simulink library "TYPEB_MASTER"  (Simulink 8.6)
settings: Solver=ode45  StartTime=0.0  StopTime=10.0  RelTol=1e-3
libraries: cdsEpicsOut x19, STATE_BIO_MASTER x17, cdsEpicsBinIn x15, cdsBit2Word x12, GAS_MASTER x12, cdsWord2Bit x5, cdsEpicsStringIn x4, cdsDacKill x4, ISC_common x4, IP_MASTER x4, cdsFilt x4, cdsEpicsMomentary x4
(part 2 of 3)

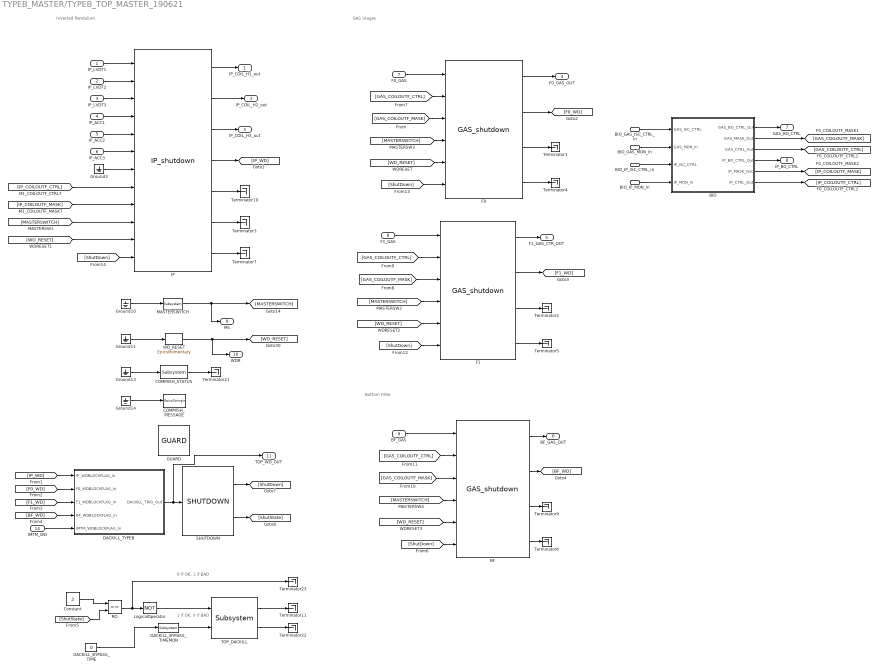
== system TYPEB_MASTER/TYPEB_TOP_MASTER_190621 ==
  note: Inverted Pendulum
  note: GAS Stages
  note: Bottom Filter
  note: 0 if OK, 1 if BAD
  note: 1 if OK, 0 if BAD
  IP_LVDT1 : Inport
  IP_LVDT2 : Inport  Port=2
  IP_LVDT3 : Inport  Port=3
  IP_ACC1 : Inport  Port=4
  IP_ACC2 : Inport  Port=5
  IP_ACC3 : Inport  Port=6
  F0_GAS : Inport  Port=7
  F1_GAS : Inport  Port=8
  BF_GAS : Inport  Port=9
  BIO_GAS_ISC_CTRL_In : Inport  Port=10
  BIO_GAS_MON_In : Inport  Port=11
  BIO_IP_ISC_CTRL_In : Inport  Port=12
  BIO_IP_MON_In : Inport  Port=13
  IMTM_WD : Inport  Port=14
  BF : GAS_MASTER/GAS_shutdown
  BIO : Subsystem
  COMMISH_MESSAGE : cdsEpicsStringIn/EpicsStringIn  Tag=cdsEpicsStringIn  Description=cdsEpicsStringIn
      settings: AttributesFormatString=%<Tag>
  COMMISH_STATUS : cdsEpicsBinIn/Subsystem  Tag=cdsEpicsBinIn  Description=|
      | Purpose:                                                                            
      | Create an EPICS binary (0 or 1) input channel to the FE realtime controls.          
      |                                                                                     
      | Operation:                                                                          
      | Outputs value from an EPICS ai record. Value is binary input (bi Epics record type).
      |                                                                                     
      | Usage:                                                                              
      | Name the part with the desired EPICS channel name.
      settings: AttributesFormatString=%<Tag>
  Constant : Constant  Value=2
  DACKILL_BYPASS_TIME : Constant  Value=0
  DACKILL_BYPASS_TIMEMON : cdsEpicsOut/Subsystem  Tag=cdsEpicsOutput  Description=|
      | Purpose:                                          
      | Output a FE signal to an EPICS channel.           
      |                                                   
      | Operation:                                        
      | Takes input value and passes it to EPICS record.  
      |                                                   
      | Usage:                                            
      | Name the part with the desired EPICS rrecord name.
      settings: AttributesFormatString=%<Tag>
  DACKILL_TYPEB : Subsystem
  F0 : GAS_MASTER/GAS_shutdown
  F1 : GAS_MASTER/GAS_shutdown
  GUARD : ISC_common/GUARD
  Ground{3,10..11,13..14} (5 alike) : Ground
  IP : IP_MASTER/IP_shutdown
  LogicalOperator : Logic  Operator=NOT  AllPortsSameDT=off  OutDataTypeStr=boolean
  MASTERSWITCH : cdsEpicsBinIn/Subsystem  Tag=cdsEpicsBinIn  Description=|
      | Purpose:                                                                            
      | Create an EPICS binary (0 or 1) input channel to the FE realtime controls.          
      |                                                                                     
      | Operation:                                                                          
      | Outputs value from an EPICS ai record. Value is binary input (bi Epics record type).
      |                                                                                     
      | Usage:                                                                              
      | Name the part with the desired EPICS channel name.
      settings: AttributesFormatString=%<Tag>
  RO : RelationalOperator  Operator===  OutDataTypeStr=boolean
  SHUTDOWN : SHUTDOWN/SHUTDOWN
  TOP_DACKILL : cdsDacKill/Subsystem  Description=cdsDacKill
      settings: AttributesFormatString=%<Description>
  Terminator{1..7,9..11,21..23} (13 alike) : Terminator
  WD_RESET : cdsEpicsMomentary/EpicsMomentary  Tag=cdsEpicsMomentary
      settings: AttributesFormatString=%<Tag>
  IP_COIL_H1_out : Outport
  IP_COIL_H2_out : Outport  Port=2
  IP_COIL_H3_out : Outport  Port=3
  F0_GAS_OUT : Outport  Port=4
  F1_GAS_CTR_OUT : Outport  Port=5
  BF_GAS_OUT : Outport  Port=6
  GAS_BO_CTRL : Outport  Port=7
  IP_BO_CTRL : Outport  Port=8
  MS : Outport  Port=9
  WDR : Outport  Port=10
  TOP_WD_OUT : Outport  Port=11
  wires:
  F1_GAS/1 -> F1/1
  [GAS_COILOUTF_MASK] -> F0/3
  [GAS_COILOUTF_CTRL] -> F0/2
  [GAS_COILOUTF_CTRL] -> BF/2
  [MASTERSWITCH] -> F0/4
  [GAS_COILOUTF_MASK] -> BF/3
  [IP_COILOUTF_CTRL] -> IP/8
  BIO/6(IP_CTRL_Out) -> [IP_COILOUTF_CTRL]
  [MASTERSWITCH] -> BF/4
  BF/1 -> BF_GAS_OUT/1
  IP_LVDT1/1 -> IP/1
  F1/1 -> F1_GAS_CTR_OUT/1
  BIO/3(GAS_CTRL_Out) -> [GAS_COILOUTF_CTRL]
  BIO/5(IP_MASK_Out) -> [IP_COILOUTF_MASK]
  F1/3 -> Terminator2/1
  LogicalOperator/1 -> TOP_DACKILL/1
  [WD_RESET] -> F1/5
  IP_LVDT2/1 -> IP/2
  [MASTERSWITCH] -> IP/10
  Ground3/1 -> IP/7
  F0/3 -> Terminator1/1
  IP/3 -> IP_COIL_H3_out/1
  BF_GAS/1 -> BF/1
  F1/2 -> [F1_WD]
  F0_GAS/1 -> F0/1
  [MASTERSWITCH] -> F1/4
  IP_LVDT3/1 -> IP/3
  IP/4 -> [IP_WD]
  [F1_WD] -> DACKILL_TYPEB/3(F1_WDBLOCKFLAG_In)
  F0/1 -> F0_GAS_OUT/1
  Ground11/1 -> WD_RESET/1
  [BF_WD] -> DACKILL_TYPEB/4(BF_WDBLOCKFLAG_In)
  IP/2 -> IP_COIL_H2_out/1
  IP/1 -> IP_COIL_H1_out/1
  Ground10/1 -> MASTERSWITCH/1
  DACKILL_BYPASS_TIME/1 -> DACKILL_BYPASS_TIMEMON/1
  F0/2 -> [F0_WD]
  IP_ACC1/1 -> IP/4
  [WD_RESET] -> BF/5
  TOP_DACKILL/1 -> Terminator11/1
  IMTM_WD/1 -> DACKILL_TYPEB/5(IMTM_WDBLOCKFLAG_In)
  [F0_WD] -> DACKILL_TYPEB/2(F0_WDBLOCKFLAG_In)
  [GAS_COILOUTF_CTRL] -> F1/2
  IP_ACC3/1 -> IP/6
  BF/2 -> [BF_WD]
  Ground14/1 -> COMMISH_MESSAGE/1
  IP/5 -> Terminator10/1
  BF/3 -> Terminator9/1
  DACKILL_BYPASS_TIMEMON/1 -> TOP_DACKILL/2
  [WD_RESET] -> IP/11
  IP_ACC2/1 -> IP/5
  [IP_WD] -> DACKILL_TYPEB/1(IP_WDBLOCKFLAG_In)
  COMMISH_STATUS/1 -> Terminator21/1
  Ground13/1 -> COMMISH_STATUS/1
  TOP_DACKILL/2 -> Terminator22/1
  BIO/4(IP_BO_CTRL_Out) -> IP_BO_CTRL/1
  BIO/1(GAS_BO_CTRL_Out) -> GAS_BO_CTRL/1
  BIO_IP_MON_In/1 -> BIO/4(IP_MON_In)
  BIO/2(GAS_MASK_Out) -> [GAS_COILOUTF_MASK]
  BIO_GAS_MON_In/1 -> BIO/2(GAS_MON_In)
  BIO_IP_ISC_CTRL_In/1 -> BIO/3(IP_ISC_CTRL)
  BIO_GAS_ISC_CTRL_In/1 -> BIO/1(GAS_ISC_CTRL)
  [IP_COILOUTF_MASK] -> IP/9
  [GAS_COILOUTF_MASK] -> F1/3
  [WD_RESET] -> F0/5
  MASTERSWITCH/1 -> MS/1, [MASTERSWITCH]
  WD_RESET/1 -> WDR/1, [WD_RESET]
  IP/6 -> Terminator3/1
  F0/4 -> Terminator4/1
  F1/4 -> Terminator5/1
  BF/4 -> Terminator6/1
  IP/7 -> Terminator7/1
  DACKILL_TYPEB/1(DACKILL_TRIG_Out) -> TOP_WD_OUT/1, SHUTDOWN/1
  SHUTDOWN/1 -> [ShutDown]
  SHUTDOWN/2 -> [ShutState]
  Constant/1 -> RO/1
  [ShutState] -> RO/2
  RO/1 -> Terminator23/1, LogicalOperator/1
  [ShutDown] -> BF/6
  [ShutDown] -> F1/6
  [ShutDown] -> F0/6
  [ShutDown] -> IP/12

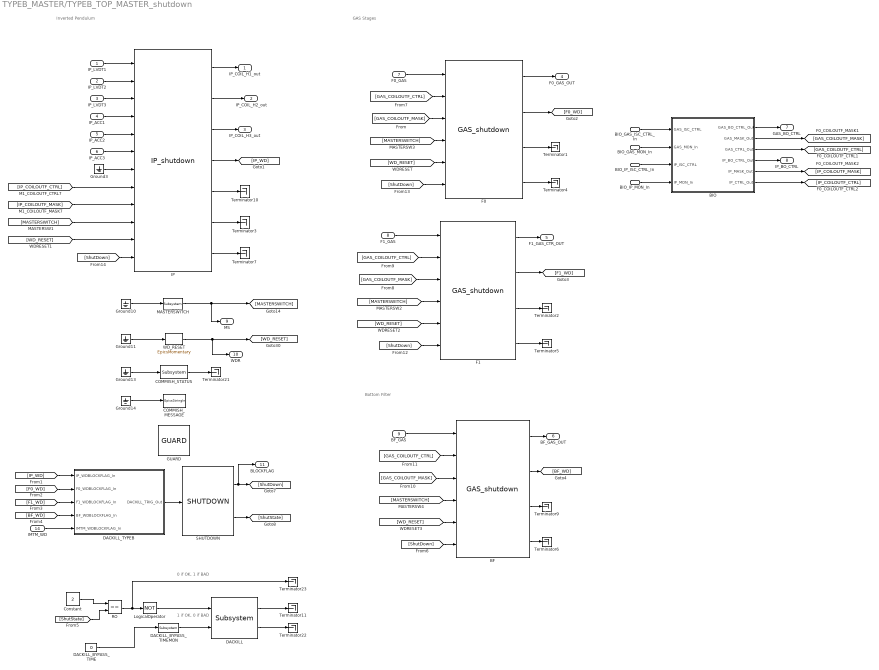
== system TYPEB_MASTER/TYPEB_TOP_MASTER_shutdown ==
  note: Inverted Pendulum
  note: GAS Stages
  note: Bottom Filter
  note: 0 if OK, 1 if BAD
  note: 1 if OK, 0 if BAD
  IP_LVDT1 : Inport
  IP_LVDT2 : Inport  Port=2
  IP_LVDT3 : Inport  Port=3
  IP_ACC1 : Inport  Port=4
  IP_ACC2 : Inport  Port=5
  IP_ACC3 : Inport  Port=6
  F0_GAS : Inport  Port=7
  F1_GAS : Inport  Port=8
  BF_GAS : Inport  Port=9
  BIO_GAS_ISC_CTRL_In : Inport  Port=10
  BIO_GAS_MON_In : Inport  Port=11
  BIO_IP_ISC_CTRL_In : Inport  Port=12
  BIO_IP_MON_In : Inport  Port=13
  IMTM_WD : Inport  Port=14
  BF : GAS_MASTER/GAS_shutdown
  BIO : Subsystem
  COMMISH_MESSAGE : cdsEpicsStringIn/EpicsStringIn  Tag=cdsEpicsStringIn  Description=cdsEpicsStringIn
      settings: AttributesFormatString=%<Tag>
  COMMISH_STATUS : cdsEpicsBinIn/Subsystem  Tag=cdsEpicsBinIn  Description=|
      | Purpose:                                                                            
      | Create an EPICS binary (0 or 1) input channel to the FE realtime controls.          
      |                                                                                     
      | Operation:                                                                          
      | Outputs value from an EPICS ai record. Value is binary input (bi Epics record type).
      |                                                                                     
      | Usage:                                                                              
      | Name the part with the desired EPICS channel name.
      settings: AttributesFormatString=%<Tag>
  Constant : Constant  Value=2
  DACKILL : cdsDacKill/Subsystem  Description=cdsDacKill
      settings: AttributesFormatString=%<Description>
  DACKILL_BYPASS_TIME : Constant  Value=0
  DACKILL_BYPASS_TIMEMON : cdsEpicsOut/Subsystem  Tag=cdsEpicsOutput  Description=|
      | Purpose:                                          
      | Output a FE signal to an EPICS channel.           
      |                                                   
      | Operation:                                        
      | Takes input value and passes it to EPICS record.  
      |                                                   
      | Usage:                                            
      | Name the part with the desired EPICS rrecord name.
      settings: AttributesFormatString=%<Tag>
  DACKILL_TYPEB : Subsystem
  F0 : GAS_MASTER/GAS_shutdown
  F1 : GAS_MASTER/GAS_shutdown
  GUARD : ISC_common/GUARD
  Ground{3,10..11,13..14} (5 alike) : Ground
  IP : IP_MASTER/IP_shutdown
  LogicalOperator : Logic  Operator=NOT  AllPortsSameDT=off  OutDataTypeStr=boolean
  MASTERSWITCH : cdsEpicsBinIn/Subsystem  Tag=cdsEpicsBinIn  Description=|
      | Purpose:                                                                            
      | Create an EPICS binary (0 or 1) input channel to the FE realtime controls.          
      |                                                                                     
      | Operation:                                                                          
      | Outputs value from an EPICS ai record. Value is binary input (bi Epics record type).
      |                                                                                     
      | Usage:                                                                              
      | Name the part with the desired EPICS channel name.
      settings: AttributesFormatString=%<Tag>
  RO : RelationalOperator  Operator===  OutDataTypeStr=boolean
  SHUTDOWN : SHUTDOWN/SHUTDOWN
  Terminator{1..7,9..11,21..23} (13 alike) : Terminator
  WD_RESET : cdsEpicsMomentary/EpicsMomentary  Tag=cdsEpicsMomentary
      settings: AttributesFormatString=%<Tag>
  IP_COIL_H1_out : Outport
  IP_COIL_H2_out : Outport  Port=2
  IP_COIL_H3_out : Outport  Port=3
  F0_GAS_OUT : Outport  Port=4
  F1_GAS_CTR_OUT : Outport  Port=5
  BF_GAS_OUT : Outport  Port=6
  GAS_BO_CTRL : Outport  Port=7
  IP_BO_CTRL : Outport  Port=8
  MS : Outport  Port=9
  WDR : Outport  Port=10
  BLOCKFLAG : Outport  Port=11
  wires:
  F1_GAS/1 -> F1/1
  [GAS_COILOUTF_MASK] -> F0/3
  [GAS_COILOUTF_CTRL] -> F0/2
  [GAS_COILOUTF_CTRL] -> BF/2
  [MASTERSWITCH] -> F0/4
  [GAS_COILOUTF_MASK] -> BF/3
  [IP_COILOUTF_CTRL] -> IP/8
  BIO/6(IP_CTRL_Out) -> [IP_COILOUTF_CTRL]
  [MASTERSWITCH] -> BF/4
  BF/1 -> BF_GAS_OUT/1
  IP_LVDT1/1 -> IP/1
  F1/1 -> F1_GAS_CTR_OUT/1
  BIO/3(GAS_CTRL_Out) -> [GAS_COILOUTF_CTRL]
  BIO/5(IP_MASK_Out) -> [IP_COILOUTF_MASK]
  F1/3 -> Terminator2/1
  LogicalOperator/1 -> DACKILL/1
  [WD_RESET] -> F1/5
  IP_LVDT2/1 -> IP/2
  [MASTERSWITCH] -> IP/10
  Ground3/1 -> IP/7
  F0/3 -> Terminator1/1
  IP/3 -> IP_COIL_H3_out/1
  BF_GAS/1 -> BF/1
  F1/2 -> [F1_WD]
  F0_GAS/1 -> F0/1
  [MASTERSWITCH] -> F1/4
  IP_LVDT3/1 -> IP/3
  IP/4 -> [IP_WD]
  [F1_WD] -> DACKILL_TYPEB/3(F1_WDBLOCKFLAG_In)
  F0/1 -> F0_GAS_OUT/1
  Ground11/1 -> WD_RESET/1
  [BF_WD] -> DACKILL_TYPEB/4(BF_WDBLOCKFLAG_In)
  IP/2 -> IP_COIL_H2_out/1
  IP/1 -> IP_COIL_H1_out/1
  Ground10/1 -> MASTERSWITCH/1
  DACKILL_BYPASS_TIME/1 -> DACKILL_BYPASS_TIMEMON/1
  F0/2 -> [F0_WD]
  IP_ACC1/1 -> IP/4
  [WD_RESET] -> BF/5
  DACKILL/1 -> Terminator11/1
  IMTM_WD/1 -> DACKILL_TYPEB/5(IMTM_WDBLOCKFLAG_In)
  [F0_WD] -> DACKILL_TYPEB/2(F0_WDBLOCKFLAG_In)
  [GAS_COILOUTF_CTRL] -> F1/2
  IP_ACC3/1 -> IP/6
  BF/2 -> [BF_WD]
  Ground14/1 -> COMMISH_MESSAGE/1
  IP/5 -> Terminator10/1
  BF/3 -> Terminator9/1
  DACKILL_BYPASS_TIMEMON/1 -> DACKILL/2
  [WD_RESET] -> IP/11
  IP_ACC2/1 -> IP/5
  [IP_WD] -> DACKILL_TYPEB/1(IP_WDBLOCKFLAG_In)
  COMMISH_STATUS/1 -> Terminator21/1
  Ground13/1 -> COMMISH_STATUS/1
  DACKILL/2 -> Terminator22/1
  BIO/4(IP_BO_CTRL_Out) -> IP_BO_CTRL/1
  BIO/1(GAS_BO_CTRL_Out) -> GAS_BO_CTRL/1
  BIO_IP_MON_In/1 -> BIO/4(IP_MON_In)
  BIO/2(GAS_MASK_Out) -> [GAS_COILOUTF_MASK]
  BIO_GAS_MON_In/1 -> BIO/2(GAS_MON_In)
  BIO_IP_ISC_CTRL_In/1 -> BIO/3(IP_ISC_CTRL)
  BIO_GAS_ISC_CTRL_In/1 -> BIO/1(GAS_ISC_CTRL)
  [IP_COILOUTF_MASK] -> IP/9
  [GAS_COILOUTF_MASK] -> F1/3
  [WD_RESET] -> F0/5
  MASTERSWITCH/1 -> MS/1, [MASTERSWITCH]
  WD_RESET/1 -> WDR/1, [WD_RESET]
  IP/6 -> Terminator3/1
  F0/4 -> Terminator4/1
  F1/4 -> Terminator5/1
  BF/4 -> Terminator6/1
  IP/7 -> Terminator7/1
  DACKILL_TYPEB/1(DACKILL_TRIG_Out) -> SHUTDOWN/1
  SHUTDOWN/1 -> BLOCKFLAG/1, [ShutDown]
  SHUTDOWN/2 -> [ShutState]
  Constant/1 -> RO/1
  [ShutState] -> RO/2
  RO/1 -> Terminator23/1, LogicalOperator/1
  [ShutDown] -> BF/6
  [ShutDown] -> F1/6
  [ShutDown] -> F0/6
  [ShutDown] -> IP/12

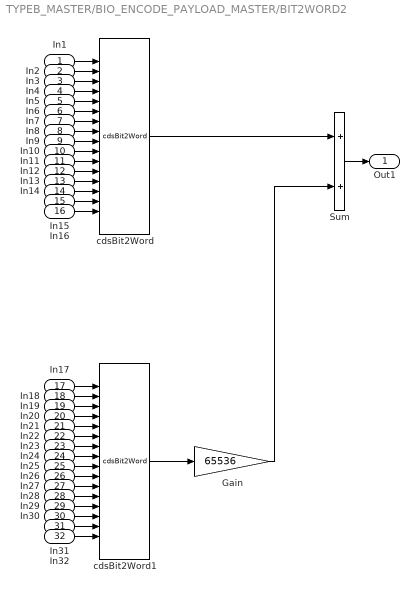
== system TYPEB_MASTER/BIO_ENCODE_PAYLOAD_MASTER/BIT2WORD2 ==
  In1 : Inport
  In2 : Inport  Port=2
  In3 : Inport  Port=3
  In4 : Inport  Port=4
  In5 : Inport  Port=5
  In6 : Inport  Port=6
  In7 : Inport  Port=7
  In8 : Inport  Port=8
  In9 : Inport  Port=9
  In10 : Inport  Port=10
  In11 : Inport  Port=11
  In12 : Inport  Port=12
  In13 : Inport  Port=13
  In14 : Inport  Port=14
  In15 : Inport  Port=15
  In16 : Inport  Port=16
  In17 : Inport  Port=17
  In18 : Inport  Port=18
  In19 : Inport  Port=19
  In20 : Inport  Port=20
  In21 : Inport  Port=21
  In22 : Inport  Port=22
  In23 : Inport  Port=23
  In24 : Inport  Port=24
  In25 : Inport  Port=25
  In26 : Inport  Port=26
  In27 : Inport  Port=27
  In28 : Inport  Port=28
  In29 : Inport  Port=29
  In30 : Inport  Port=30
  In31 : Inport  Port=31
  In32 : Inport  Port=32
  Gain : Gain  Gain=65536
  Sum : Sum
  cdsBit2Word : cdsBit2Word/cdsBit2Word  Tag=cdsBit2Word  Description=Forms single 16 bit integer from 16 0/1 inputs.
      settings: AttributesFormatString=%<Tag>
  cdsBit2Word1 : cdsBit2Word/cdsBit2Word  Tag=cdsBit2Word  Description=Forms single 16 bit integer from 16 0/1 inputs.
      settings: AttributesFormatString=%<Tag>
  Out1 : Outport
  wires:
  Gain/1 -> Sum/2
  cdsBit2Word1/1 -> Gain/1
  cdsBit2Word/1 -> Sum/1
  In1/1 -> cdsBit2Word/1
  In2/1 -> cdsBit2Word/2
  In3/1 -> cdsBit2Word/3
  In4/1 -> cdsBit2Word/4
  In5/1 -> cdsBit2Word/5
  In6/1 -> cdsBit2Word/6
  In7/1 -> cdsBit2Word/7
  In8/1 -> cdsBit2Word/8
  In9/1 -> cdsBit2Word/9
  In10/1 -> cdsBit2Word/10
  Sum/1 -> Out1/1
  In11/1 -> cdsBit2Word/11
  In12/1 -> cdsBit2Word/12
  In13/1 -> cdsBit2Word/13
  In14/1 -> cdsBit2Word/14
  In15/1 -> cdsBit2Word/15
  In16/1 -> cdsBit2Word/16
  In17/1 -> cdsBit2Word1/1
  In18/1 -> cdsBit2Word1/2
  In19/1 -> cdsBit2Word1/3
  In20/1 -> cdsBit2Word1/4
  In21/1 -> cdsBit2Word1/5
  In22/1 -> cdsBit2Word1/6
  In23/1 -> cdsBit2Word1/7
  In24/1 -> cdsBit2Word1/8
  In25/1 -> cdsBit2Word1/9
  In26/1 -> cdsBit2Word1/10
  In27/1 -> cdsBit2Word1/11
  In28/1 -> cdsBit2Word1/12
  In29/1 -> cdsBit2Word1/13
  In30/1 -> cdsBit2Word1/14
  In31/1 -> cdsBit2Word1/15
  In32/1 -> cdsBit2Word1/16

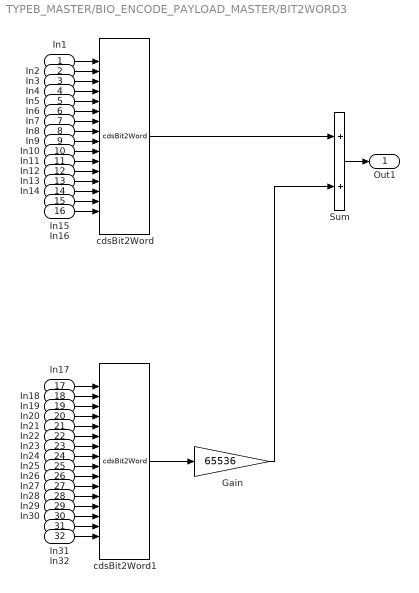
== system TYPEB_MASTER/BIO_ENCODE_PAYLOAD_MASTER/BIT2WORD3 ==
  In1 : Inport
  In2 : Inport  Port=2
  In3 : Inport  Port=3
  In4 : Inport  Port=4
  In5 : Inport  Port=5
  In6 : Inport  Port=6
  In7 : Inport  Port=7
  In8 : Inport  Port=8
  In9 : Inport  Port=9
  In10 : Inport  Port=10
  In11 : Inport  Port=11
  In12 : Inport  Port=12
  In13 : Inport  Port=13
  In14 : Inport  Port=14
  In15 : Inport  Port=15
  In16 : Inport  Port=16
  In17 : Inport  Port=17
  In18 : Inport  Port=18
  In19 : Inport  Port=19
  In20 : Inport  Port=20
  In21 : Inport  Port=21
  In22 : Inport  Port=22
  In23 : Inport  Port=23
  In24 : Inport  Port=24
  In25 : Inport  Port=25
  In26 : Inport  Port=26
  In27 : Inport  Port=27
  In28 : Inport  Port=28
  In29 : Inport  Port=29
  In30 : Inport  Port=30
  In31 : Inport  Port=31
  In32 : Inport  Port=32
  Gain : Gain  Gain=65536
  Sum : Sum
  cdsBit2Word : cdsBit2Word/cdsBit2Word  Tag=cdsBit2Word  Description=Forms single 16 bit integer from 16 0/1 inputs.
      settings: AttributesFormatString=%<Tag>
  cdsBit2Word1 : cdsBit2Word/cdsBit2Word  Tag=cdsBit2Word  Description=Forms single 16 bit integer from 16 0/1 inputs.
      settings: AttributesFormatString=%<Tag>
  Out1 : Outport
  wires:
  Gain/1 -> Sum/2
  cdsBit2Word1/1 -> Gain/1
  cdsBit2Word/1 -> Sum/1
  In1/1 -> cdsBit2Word/1
  In2/1 -> cdsBit2Word/2
  In3/1 -> cdsBit2Word/3
  In4/1 -> cdsBit2Word/4
  In5/1 -> cdsBit2Word/5
  In6/1 -> cdsBit2Word/6
  In7/1 -> cdsBit2Word/7
  In8/1 -> cdsBit2Word/8
  In9/1 -> cdsBit2Word/9
  In10/1 -> cdsBit2Word/10
  Sum/1 -> Out1/1
  In11/1 -> cdsBit2Word/11
  In12/1 -> cdsBit2Word/12
  In13/1 -> cdsBit2Word/13
  In14/1 -> cdsBit2Word/14
  In15/1 -> cdsBit2Word/15
  In16/1 -> cdsBit2Word/16
  In17/1 -> cdsBit2Word1/1
  In18/1 -> cdsBit2Word1/2
  In19/1 -> cdsBit2Word1/3
  In20/1 -> cdsBit2Word1/4
  In21/1 -> cdsBit2Word1/5
  In22/1 -> cdsBit2Word1/6
  In23/1 -> cdsBit2Word1/7
  In24/1 -> cdsBit2Word1/8
  In25/1 -> cdsBit2Word1/9
  In26/1 -> cdsBit2Word1/10
  In27/1 -> cdsBit2Word1/11
  In28/1 -> cdsBit2Word1/12
  In29/1 -> cdsBit2Word1/13
  In30/1 -> cdsBit2Word1/14
  In31/1 -> cdsBit2Word1/15
  In32/1 -> cdsBit2Word1/16

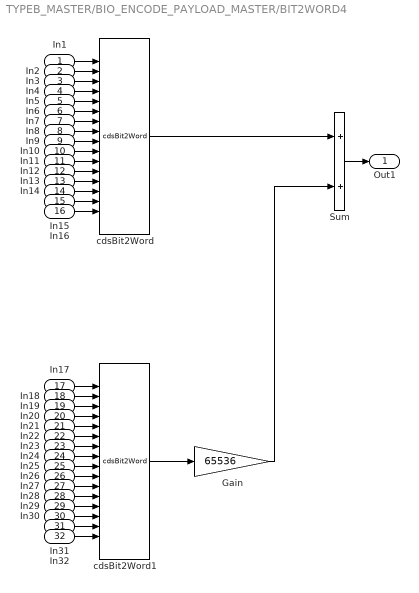
== system TYPEB_MASTER/BIO_ENCODE_PAYLOAD_MASTER/BIT2WORD4 ==
  In1 : Inport
  In2 : Inport  Port=2
  In3 : Inport  Port=3
  In4 : Inport  Port=4
  In5 : Inport  Port=5
  In6 : Inport  Port=6
  In7 : Inport  Port=7
  In8 : Inport  Port=8
  In9 : Inport  Port=9
  In10 : Inport  Port=10
  In11 : Inport  Port=11
  In12 : Inport  Port=12
  In13 : Inport  Port=13
  In14 : Inport  Port=14
  In15 : Inport  Port=15
  In16 : Inport  Port=16
  In17 : Inport  Port=17
  In18 : Inport  Port=18
  In19 : Inport  Port=19
  In20 : Inport  Port=20
  In21 : Inport  Port=21
  In22 : Inport  Port=22
  In23 : Inport  Port=23
  In24 : Inport  Port=24
  In25 : Inport  Port=25
  In26 : Inport  Port=26
  In27 : Inport  Port=27
  In28 : Inport  Port=28
  In29 : Inport  Port=29
  In30 : Inport  Port=30
  In31 : Inport  Port=31
  In32 : Inport  Port=32
  Gain : Gain  Gain=65536
  Sum : Sum
  cdsBit2Word : cdsBit2Word/cdsBit2Word  Tag=cdsBit2Word  Description=Forms single 16 bit integer from 16 0/1 inputs.
      settings: AttributesFormatString=%<Tag>
  cdsBit2Word1 : cdsBit2Word/cdsBit2Word  Tag=cdsBit2Word  Description=Forms single 16 bit integer from 16 0/1 inputs.
      settings: AttributesFormatString=%<Tag>
  Out1 : Outport
  wires:
  Gain/1 -> Sum/2
  cdsBit2Word1/1 -> Gain/1
  cdsBit2Word/1 -> Sum/1
  In1/1 -> cdsBit2Word/1
  In2/1 -> cdsBit2Word/2
  In3/1 -> cdsBit2Word/3
  In4/1 -> cdsBit2Word/4
  In5/1 -> cdsBit2Word/5
  In6/1 -> cdsBit2Word/6
  In7/1 -> cdsBit2Word/7
  In8/1 -> cdsBit2Word/8
  In9/1 -> cdsBit2Word/9
  In10/1 -> cdsBit2Word/10
  Sum/1 -> Out1/1
  In11/1 -> cdsBit2Word/11
  In12/1 -> cdsBit2Word/12
  In13/1 -> cdsBit2Word/13
  In14/1 -> cdsBit2Word/14
  In15/1 -> cdsBit2Word/15
  In16/1 -> cdsBit2Word/16
  In17/1 -> cdsBit2Word1/1
  In18/1 -> cdsBit2Word1/2
  In19/1 -> cdsBit2Word1/3
  In20/1 -> cdsBit2Word1/4
  In21/1 -> cdsBit2Word1/5
  In22/1 -> cdsBit2Word1/6
  In23/1 -> cdsBit2Word1/7
  In24/1 -> cdsBit2Word1/8
  In25/1 -> cdsBit2Word1/9
  In26/1 -> cdsBit2Word1/10
  In27/1 -> cdsBit2Word1/11
  In28/1 -> cdsBit2Word1/12
  In29/1 -> cdsBit2Word1/13
  In30/1 -> cdsBit2Word1/14
  In31/1 -> cdsBit2Word1/15
  In32/1 -> cdsBit2Word1/16

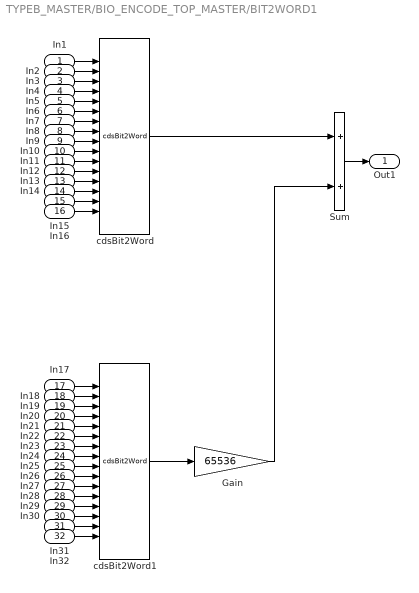
== system TYPEB_MASTER/BIO_ENCODE_TOP_MASTER/BIT2WORD1 ==
  In1 : Inport
  In2 : Inport  Port=2
  In3 : Inport  Port=3
  In4 : Inport  Port=4
  In5 : Inport  Port=5
  In6 : Inport  Port=6
  In7 : Inport  Port=7
  In8 : Inport  Port=8
  In9 : Inport  Port=9
  In10 : Inport  Port=10
  In11 : Inport  Port=11
  In12 : Inport  Port=12
  In13 : Inport  Port=13
  In14 : Inport  Port=14
  In15 : Inport  Port=15
  In16 : Inport  Port=16
  In17 : Inport  Port=17
  In18 : Inport  Port=18
  In19 : Inport  Port=19
  In20 : Inport  Port=20
  In21 : Inport  Port=21
  In22 : Inport  Port=22
  In23 : Inport  Port=23
  In24 : Inport  Port=24
  In25 : Inport  Port=25
  In26 : Inport  Port=26
  In27 : Inport  Port=27
  In28 : Inport  Port=28
  In29 : Inport  Port=29
  In30 : Inport  Port=30
  In31 : Inport  Port=31
  In32 : Inport  Port=32
  Gain : Gain  Gain=65536
  Sum : Sum
  cdsBit2Word : cdsBit2Word/cdsBit2Word  Tag=cdsBit2Word  Description=Forms single 16 bit integer from 16 0/1 inputs.
      settings: AttributesFormatString=%<Tag>
  cdsBit2Word1 : cdsBit2Word/cdsBit2Word  Tag=cdsBit2Word  Description=Forms single 16 bit integer from 16 0/1 inputs.
      settings: AttributesFormatString=%<Tag>
  Out1 : Outport
  wires:
  Gain/1 -> Sum/2
  cdsBit2Word1/1 -> Gain/1
  cdsBit2Word/1 -> Sum/1
  In1/1 -> cdsBit2Word/1
  In2/1 -> cdsBit2Word/2
  In3/1 -> cdsBit2Word/3
  In4/1 -> cdsBit2Word/4
  In5/1 -> cdsBit2Word/5
  In6/1 -> cdsBit2Word/6
  In7/1 -> cdsBit2Word/7
  In8/1 -> cdsBit2Word/8
  In9/1 -> cdsBit2Word/9
  In10/1 -> cdsBit2Word/10
  Sum/1 -> Out1/1
  In11/1 -> cdsBit2Word/11
  In12/1 -> cdsBit2Word/12
  In13/1 -> cdsBit2Word/13
  In14/1 -> cdsBit2Word/14
  In15/1 -> cdsBit2Word/15
  In16/1 -> cdsBit2Word/16
  In17/1 -> cdsBit2Word1/1
  In18/1 -> cdsBit2Word1/2
  In19/1 -> cdsBit2Word1/3
  In20/1 -> cdsBit2Word1/4
  In21/1 -> cdsBit2Word1/5
  In22/1 -> cdsBit2Word1/6
  In23/1 -> cdsBit2Word1/7
  In24/1 -> cdsBit2Word1/8
  In25/1 -> cdsBit2Word1/9
  In26/1 -> cdsBit2Word1/10
  In27/1 -> cdsBit2Word1/11
  In28/1 -> cdsBit2Word1/12
  In29/1 -> cdsBit2Word1/13
  In30/1 -> cdsBit2Word1/14
  In31/1 -> cdsBit2Word1/15
  In32/1 -> cdsBit2Word1/16

== system TYPEB_MASTER/BIO_ENCODE_TOP_MASTER/BIT2WORD2 ==
  In1 : Inport
  In2 : Inport  Port=2
  In3 : Inport  Port=3
  In4 : Inport  Port=4
  In5 : Inport  Port=5
  In6 : Inport  Port=6
  In7 : Inport  Port=7
  In8 : Inport  Port=8
  In9 : Inport  Port=9
  In10 : Inport  Port=10
  In11 : Inport  Port=11
  In12 : Inport  Port=12
  In13 : Inport  Port=13
  In14 : Inport  Port=14
  In15 : Inport  Port=15
  In16 : Inport  Port=16
  In17 : Inport  Port=17
  In18 : Inport  Port=18
  In19 : Inport  Port=19
  In20 : Inport  Port=20
  In21 : Inport  Port=21
  In22 : Inport  Port=22
  In23 : Inport  Port=23
  In24 : Inport  Port=24
  In25 : Inport  Port=25
  In26 : Inport  Port=26
  In27 : Inport  Port=27
  In28 : Inport  Port=28
  In29 : Inport  Port=29
  In30 : Inport  Port=30
  In31 : Inport  Port=31
  In32 : Inport  Port=32
  Gain : Gain  Gain=65536
  Sum : Sum
  cdsBit2Word : cdsBit2Word/cdsBit2Word  Tag=cdsBit2Word  Description=Forms single 16 bit integer from 16 0/1 inputs.
      settings: AttributesFormatString=%<Tag>
  cdsBit2Word1 : cdsBit2Word/cdsBit2Word  Tag=cdsBit2Word  Description=Forms single 16 bit integer from 16 0/1 inputs.
      settings: AttributesFormatString=%<Tag>
  Out1 : Outport
  wires:
  Gain/1 -> Sum/2
  cdsBit2Word1/1 -> Gain/1
  cdsBit2Word/1 -> Sum/1
  In1/1 -> cdsBit2Word/1
  In2/1 -> cdsBit2Word/2
  In3/1 -> cdsBit2Word/3
  In4/1 -> cdsBit2Word/4
  In5/1 -> cdsBit2Word/5
  In6/1 -> cdsBit2Word/6
  In7/1 -> cdsBit2Word/7
  In8/1 -> cdsBit2Word/8
  In9/1 -> cdsBit2Word/9
  In10/1 -> cdsBit2Word/10
  Sum/1 -> Out1/1
  In11/1 -> cdsBit2Word/11
  In12/1 -> cdsBit2Word/12
  In13/1 -> cdsBit2Word/13
  In14/1 -> cdsBit2Word/14
  In15/1 -> cdsBit2Word/15
  In16/1 -> cdsBit2Word/16
  In17/1 -> cdsBit2Word1/1
  In18/1 -> cdsBit2Word1/2
  In19/1 -> cdsBit2Word1/3
  In20/1 -> cdsBit2Word1/4
  In21/1 -> cdsBit2Word1/5
  In22/1 -> cdsBit2Word1/6
  In23/1 -> cdsBit2Word1/7
  In24/1 -> cdsBit2Word1/8
  In25/1 -> cdsBit2Word1/9
  In26/1 -> cdsBit2Word1/10
  In27/1 -> cdsBit2Word1/11
  In28/1 -> cdsBit2Word1/12
  In29/1 -> cdsBit2Word1/13
  In30/1 -> cdsBit2Word1/14
  In31/1 -> cdsBit2Word1/15
  In32/1 -> cdsBit2Word1/16

== system TYPEB_MASTER/BIO_ENCODE_TOP_MASTER/BIT2WORD5 ==
  In1 : Inport
  In2 : Inport  Port=2
  In3 : Inport  Port=3
  In4 : Inport  Port=4
  In5 : Inport  Port=5
  In6 : Inport  Port=6
  In7 : Inport  Port=7
  In8 : Inport  Port=8
  In9 : Inport  Port=9
  In10 : Inport  Port=10
  In11 : Inport  Port=11
  In12 : Inport  Port=12
  In13 : Inport  Port=13
  In14 : Inport  Port=14
  In15 : Inport  Port=15
  In16 : Inport  Port=16
  In17 : Inport  Port=17
  In18 : Inport  Port=18
  In19 : Inport  Port=19
  In20 : Inport  Port=20
  In21 : Inport  Port=21
  In22 : Inport  Port=22
  In23 : Inport  Port=23
  In24 : Inport  Port=24
  In25 : Inport  Port=25
  In26 : Inport  Port=26
  In27 : Inport  Port=27
  In28 : Inport  Port=28
  In29 : Inport  Port=29
  In30 : Inport  Port=30
  In31 : Inport  Port=31
  In32 : Inport  Port=32
  Gain : Gain  Gain=65536
  Sum : Sum
  cdsBit2Word : cdsBit2Word/cdsBit2Word  Tag=cdsBit2Word  Description=Forms single 16 bit integer from 16 0/1 inputs.
      settings: AttributesFormatString=%<Tag>
  cdsBit2Word1 : cdsBit2Word/cdsBit2Word  Tag=cdsBit2Word  Description=Forms single 16 bit integer from 16 0/1 inputs.
      settings: AttributesFormatString=%<Tag>
  Out1 : Outport
  wires:
  Gain/1 -> Sum/2
  cdsBit2Word1/1 -> Gain/1
  cdsBit2Word/1 -> Sum/1
  In1/1 -> cdsBit2Word/1
  In2/1 -> cdsBit2Word/2
  In3/1 -> cdsBit2Word/3
  In4/1 -> cdsBit2Word/4
  In5/1 -> cdsBit2Word/5
  In6/1 -> cdsBit2Word/6
  In7/1 -> cdsBit2Word/7
  In8/1 -> cdsBit2Word/8
  In9/1 -> cdsBit2Word/9
  In10/1 -> cdsBit2Word/10
  Sum/1 -> Out1/1
  In11/1 -> cdsBit2Word/11
  In12/1 -> cdsBit2Word/12
  In13/1 -> cdsBit2Word/13
  In14/1 -> cdsBit2Word/14
  In15/1 -> cdsBit2Word/15
  In16/1 -> cdsBit2Word/16
  In17/1 -> cdsBit2Word1/1
  In18/1 -> cdsBit2Word1/2
  In19/1 -> cdsBit2Word1/3
  In20/1 -> cdsBit2Word1/4
  In21/1 -> cdsBit2Word1/5
  In22/1 -> cdsBit2Word1/6
  In23/1 -> cdsBit2Word1/7
  In24/1 -> cdsBit2Word1/8
  In25/1 -> cdsBit2Word1/9
  In26/1 -> cdsBit2Word1/10
  In27/1 -> cdsBit2Word1/11
  In28/1 -> cdsBit2Word1/12
  In29/1 -> cdsBit2Word1/13
  In30/1 -> cdsBit2Word1/14
  In31/1 -> cdsBit2Word1/15
  In32/1 -> cdsBit2Word1/16

== system TYPEB_MASTER/TYPEB_MASTER/BIO ==
  note: 12 Bit Word
  note: 12 Bit Word
  note: 12 Bit Word
  note: 12 Bit Word
  TM_ISC_CTRL : Inport
  TM_MON_In : Inport  Port=2
  IM1_CTRL : Inport  Port=3
  IM1_MON_In : Inport  Port=4
  IM2_ISC_CTRL : Inport  Port=5
  IM2_MON_In : Inport  Port=6
  GAS_ISC_CTRL : Inport  Port=7
  GAS_MON_In : Inport  Port=8
  IP_ISC_CTRL : Inport  Port=9
  IP_MON_In : Inport  Port=10
  GAS : STATE_BIO_MASTER/UIM_BIO_MASTER
  IM1 : STATE_BIO_MASTER/UIM_BIO_MASTER
  IM2 : STATE_BIO_MASTER/UIM_BIO_MASTER
  IP : STATE_BIO_MASTER/TACQ_BIO_MASTER
  TM : STATE_BIO_MASTER/UIM_BIO_MASTER
  TM_BO_CTRL_Out : Outport
  TM_MASK_Out : Outport  Port=2
  TM_CTRL_Out : Outport  Port=3
  IM1_BO_CTRL_Out : Outport  Port=4
  IM1_MASK_Out : Outport  Port=5
  IM1_CTRL_Out : Outport  Port=6
  IM2_BO_CTRL_Out : Outport  Port=7
  IM2_MASK_Out : Outport  Port=8
  IM2_CTRL_Out : Outport  Port=9
  GAS_BO_CTRL_Out : Outport  Port=10
  GAS_MASK_Out : Outport  Port=11
  GAS_CTRL_Out : Outport  Port=12
  IP_BO_CTRL_Out : Outport  Port=13
  IP_MASK_Out : Outport  Port=14
  IP_CTRL_Out : Outport  Port=15
  wires:
  TM_MON_In/1 -> TM/2
  TM_ISC_CTRL/1 -> TM/1
  IM1_CTRL/1 -> IM1/1
  IM1_MON_In/1 -> IM1/2
  IM2_MON_In/1 -> IM2/2
  IM2_ISC_CTRL/1 -> IM2/1
  GAS_MON_In/1 -> GAS/2
  GAS_ISC_CTRL/1 -> GAS/1
  IP_MON_In/1 -> IP/2
  IP_ISC_CTRL/1 -> IP/1
  TM/1 -> TM_MASK_Out/1
  TM/2 -> TM_CTRL_Out/1
  TM/3 -> TM_BO_CTRL_Out/1
  IM1/1 -> IM1_MASK_Out/1
  IM1/2 -> IM1_CTRL_Out/1
  IM1/3 -> IM1_BO_CTRL_Out/1
  IM2/1 -> IM2_MASK_Out/1
  IM2/2 -> IM2_CTRL_Out/1
  IM2/3 -> IM2_BO_CTRL_Out/1
  GAS/1 -> GAS_MASK_Out/1
  GAS/2 -> GAS_CTRL_Out/1
  GAS/3 -> GAS_BO_CTRL_Out/1
  IP/1 -> IP_MASK_Out/1
  IP/2 -> IP_CTRL_Out/1
  IP/3 -> IP_BO_CTRL_Out/1

== system TYPEB_MASTER/TYPEB_MASTER/TM_OSEM ==
  OSEM_H1_In : Inport
  OSEM_H2_In : Inport  Port=2
  OSEM_H3_In : Inport  Port=3
  OSEM_H4_In : Inport  Port=4
  2EUL : cdsMuxMatrix/Subsystem  Tag=cdsMuxMatrix  Description=Any size matrix. Inputs and outputs must be connected using Mux and Demux parts.
      settings: AttributesFormatString=%<Tag>
  DAMP : Subsystem  AncestorBlock=SIXOSEM_F_STAGE_MASTER/SIXOSEM_F_STAGE_MASTER/DAMP
  Demux1 : Demux  Outputs=3
  Demux2 : Demux  Outputs=3
  INF : Subsystem  AncestorBlock=SIXOSEM_F_STAGE_MASTER/SIXOSEM_F_STAGE_MASTER/OSEMINF
  Mux1 : Mux  Inputs=3
  Mux2 : Mux
  SENSALIGN : cdsMuxMatrix/Subsystem  Tag=cdsMuxMatrix  Description=Any size matrix. Inputs and outputs must be connected using Mux and Demux parts.
      settings: AttributesFormatString=%<Tag>
  wires:
  Mux1/1 -> SENSALIGN/1
  SENSALIGN/1 -> Demux2/1
  Demux1/3 -> Mux1/3
  Mux2/1 -> 2EUL/1
  2EUL/1 -> Demux1/1
  Demux1/1 -> Mux1/1
  Demux1/2 -> Mux1/2
  OSEM_H1_In/1 -> INF/1(H1_In)
  OSEM_H4_In/1 -> INF/4(H4_In)
  OSEM_H3_In/1 -> INF/3(H3_In)
  OSEM_H2_In/1 -> INF/2(H2_In)
  Demux2/1 -> DAMP/1(LONG_In)
  Demux2/2 -> DAMP/2(PITCH_In)
  Demux2/3 -> DAMP/3(YAW_In)
  INF/1(H4_Out) -> Mux2/1
  INF/2(H1_Out) -> Mux2/2
  INF/3(H2_Out) -> Mux2/3
  INF/4(H3_Out) -> Mux2/4

== system TYPEB_MASTER/TYPEB_PAYLOAD_MASTER/BIO ==
  note: 12 Bit Word
  note: 12 Bit Word
  TM_ISC_CTRL : Inport
  TM_MON_In : Inport  Port=2
  IMV_CTRL : Inport  Port=3
  IMV_MON_In : Inport  Port=4
  IMH_ISC_CTRL : Inport  Port=5
  IMH_MON_In : Inport  Port=6
  IMH : STATE_BIO_MASTER/UIM_BIO_MASTER
  IMV : STATE_BIO_MASTER/UIM_BIO_MASTER
  TM : STATE_BIO_MASTER/UIM_BIO_MASTER
  TM_BO_CTRL_Out : Outport
  TM_MASK_Out : Outport  Port=2
  TM_CTRL_Out : Outport  Port=3
  IMV_BO_CTRL_Out : Outport  Port=4
  IMV_MASK_Out : Outport  Port=5
  IMV_CTRL_Out : Outport  Port=6
  IMH_BO_CTRL_Out : Outport  Port=7
  IMH_MASK_Out : Outport  Port=8
  IMH_CTRL_Out : Outport  Port=9
  wires:
  IMH/3 -> IMH_BO_CTRL_Out/1
  IMH/2 -> IMH_CTRL_Out/1
  IMH/1 -> IMH_MASK_Out/1
  IMV/3 -> IMV_BO_CTRL_Out/1
  IMV/1 -> IMV_MASK_Out/1
  IMV/2 -> IMV_CTRL_Out/1
  TM/2 -> TM_CTRL_Out/1
  TM/3 -> TM_BO_CTRL_Out/1
  TM/1 -> TM_MASK_Out/1
  IMH_ISC_CTRL/1 -> IMH/1
  IMV_MON_In/1 -> IMV/2
  IMH_MON_In/1 -> IMH/2
  TM_ISC_CTRL/1 -> TM/1
  IMV_CTRL/1 -> IMV/1
  TM_MON_In/1 -> TM/2

== system TYPEB_MASTER/TYPEB_PAYLOAD_shutdown/BIO ==
  note: 12 Bit Word
  note: 12 Bit Word
  TM_ISC_CTRL : Inport
  TM_MON_In : Inport  Port=2
  IMV_CTRL : Inport  Port=3
  IMV_MON_In : Inport  Port=4
  IMH_ISC_CTRL : Inport  Port=5
  IMH_MON_In : Inport  Port=6
  IMH : STATE_BIO_MASTER/UIM_BIO_MASTER
  IMV : STATE_BIO_MASTER/UIM_BIO_MASTER
  TM : STATE_BIO_MASTER/UIM_BIO_MASTER
  TM_BO_CTRL_Out : Outport
  TM_MASK_Out : Outport  Port=2
  TM_CTRL_Out : Outport  Port=3
  IMV_BO_CTRL_Out : Outport  Port=4
  IMV_MASK_Out : Outport  Port=5
  IMV_CTRL_Out : Outport  Port=6
  IMH_BO_CTRL_Out : Outport  Port=7
  IMH_MASK_Out : Outport  Port=8
  IMH_CTRL_Out : Outport  Port=9
  wires:
  TM_MON_In/1 -> TM/2
  IMV_CTRL/1 -> IMV/1
  TM_ISC_CTRL/1 -> TM/1
  IMH_MON_In/1 -> IMH/2
  IMV_MON_In/1 -> IMV/2
  IMH_ISC_CTRL/1 -> IMH/1
  TM/1 -> TM_MASK_Out/1
  TM/3 -> TM_BO_CTRL_Out/1
  TM/2 -> TM_CTRL_Out/1
  IMV/2 -> IMV_CTRL_Out/1
  IMV/1 -> IMV_MASK_Out/1
  IMV/3 -> IMV_BO_CTRL_Out/1
  IMH/1 -> IMH_MASK_Out/1
  IMH/2 -> IMH_CTRL_Out/1
  IMH/3 -> IMH_BO_CTRL_Out/1

== system TYPEB_MASTER/TYPEB_TOP_MASTER/BIO ==
  note: 12 Bit Word
  note: 12 Bit Word
  GAS_ISC_CTRL : Inport
  GAS_MON_In : Inport  Port=2
  IP_ISC_CTRL : Inport  Port=3
  IP_MON_In : Inport  Port=4
  GAS : STATE_BIO_MASTER/UIM_BIO_MASTER
  IP : STATE_BIO_MASTER/TACQ_BIO_MASTER
  GAS_BO_CTRL_Out : Outport
  GAS_MASK_Out : Outport  Port=2
  GAS_CTRL_Out : Outport  Port=3
  IP_BO_CTRL_Out : Outport  Port=4
  IP_MASK_Out : Outport  Port=5
  IP_CTRL_Out : Outport  Port=6
  wires:
  IP/2 -> IP_CTRL_Out/1
  GAS/1 -> GAS_MASK_Out/1
  IP_MON_In/1 -> IP/2
  IP/3 -> IP_BO_CTRL_Out/1
  GAS/2 -> GAS_CTRL_Out/1
  GAS/3 -> GAS_BO_CTRL_Out/1
  GAS_MON_In/1 -> GAS/2
  GAS_ISC_CTRL/1 -> GAS/1
  IP/1 -> IP_MASK_Out/1
  IP_ISC_CTRL/1 -> IP/1

== system TYPEB_MASTER/TYPEB_TOP_MASTER/DACKILL_TYPEB ==
  note: AND is zero  (0) if all stages are OK
      | non-zero if BAD
  note: WDBLOCKFLAG is zero (0) if OK,
      | non-zero if BAD
  IP_WDBLOCKFLAG_In : Inport
  F0_WDBLOCKFLAG_In : Inport  Port=2
  F1_WDBLOCKFLAG_In : Inport  Port=3
  BF_WDBLOCKFLAG_In : Inport  Port=4
  IMTM_WDBLOCKFLAG_In : Inport  Port=5
  LogicalOperator1 : Logic  Operator=OR  Inputs=5  AllPortsSameDT=off  OutDataTypeStr=boolean
  STATE : cdsEpicsOut/Subsystem  Tag=cdsEpicsOutput  Description=|
      | Purpose:                                          
      | Output a FE signal to an EPICS channel.           
      |                                                   
      | Operation:                                        
      | Takes input value and passes it to EPICS record.  
      |                                                   
      | Usage:                                            
      | Name the part with the desired EPICS rrecord name.
      settings: AttributesFormatString=%<Tag>
  DACKILL_TRIG_Out : Outport
  wires:
  BF_WDBLOCKFLAG_In/1 -> LogicalOperator1/4
  IMTM_WDBLOCKFLAG_In/1 -> LogicalOperator1/5
  LogicalOperator1/1 -> STATE/1
  F1_WDBLOCKFLAG_In/1 -> LogicalOperator1/3
  F0_WDBLOCKFLAG_In/1 -> LogicalOperator1/2
  IP_WDBLOCKFLAG_In/1 -> LogicalOperator1/1
  STATE/1 -> DACKILL_TRIG_Out/1

== system TYPEB_MASTER/TYPEB_TOP_MASTER_190621/BIO ==
  note: 12 Bit Word
  note: 12 Bit Word
  GAS_ISC_CTRL : Inport
  GAS_MON_In : Inport  Port=2
  IP_ISC_CTRL : Inport  Port=3
  IP_MON_In : Inport  Port=4
  GAS : STATE_BIO_MASTER/UIM_BIO_MASTER
  IP : STATE_BIO_MASTER/TACQ_BIO_MASTER
  GAS_BO_CTRL_Out : Outport
  GAS_MASK_Out : Outport  Port=2
  GAS_CTRL_Out : Outport  Port=3
  IP_BO_CTRL_Out : Outport  Port=4
  IP_MASK_Out : Outport  Port=5
  IP_CTRL_Out : Outport  Port=6
  wires:
  IP/2 -> IP_CTRL_Out/1
  GAS/1 -> GAS_MASK_Out/1
  IP_MON_In/1 -> IP/2
  IP/3 -> IP_BO_CTRL_Out/1
  GAS/2 -> GAS_CTRL_Out/1
  GAS/3 -> GAS_BO_CTRL_Out/1
  GAS_MON_In/1 -> GAS/2
  GAS_ISC_CTRL/1 -> GAS/1
  IP/1 -> IP_MASK_Out/1
  IP_ISC_CTRL/1 -> IP/1

== system TYPEB_MASTER/TYPEB_TOP_MASTER_190621/DACKILL_TYPEB ==
  note: AND is zero  (0) if all stages are OK
      | non-zero if BAD
  note: WDBLOCKFLAG is zero (0) if OK,
      | non-zero if BAD
  IP_WDBLOCKFLAG_In : Inport
  F0_WDBLOCKFLAG_In : Inport  Port=2
  F1_WDBLOCKFLAG_In : Inport  Port=3
  BF_WDBLOCKFLAG_In : Inport  Port=4
  IMTM_WDBLOCKFLAG_In : Inport  Port=5
  LogicalOperator1 : Logic  Operator=OR  Inputs=5  AllPortsSameDT=off  OutDataTypeStr=boolean
  STATE : cdsEpicsOut/Subsystem  Tag=cdsEpicsOutput  Description=|
      | Purpose:                                          
      | Output a FE signal to an EPICS channel.           
      |                                                   
      | Operation:                                        
      | Takes input value and passes it to EPICS record.  
      |                                                   
      | Usage:                                            
      | Name the part with the desired EPICS rrecord name.
      settings: AttributesFormatString=%<Tag>
  DACKILL_TRIG_Out : Outport
  wires:
  BF_WDBLOCKFLAG_In/1 -> LogicalOperator1/4
  IMTM_WDBLOCKFLAG_In/1 -> LogicalOperator1/5
  LogicalOperator1/1 -> STATE/1
  F1_WDBLOCKFLAG_In/1 -> LogicalOperator1/3
  F0_WDBLOCKFLAG_In/1 -> LogicalOperator1/2
  IP_WDBLOCKFLAG_In/1 -> LogicalOperator1/1
  STATE/1 -> DACKILL_TRIG_Out/1

== system TYPEB_MASTER/TYPEB_TOP_MASTER_shutdown/BIO ==
  note: 12 Bit Word
  note: 12 Bit Word
  GAS_ISC_CTRL : Inport
  GAS_MON_In : Inport  Port=2
  IP_ISC_CTRL : Inport  Port=3
  IP_MON_In : Inport  Port=4
  GAS : STATE_BIO_MASTER/UIM_BIO_MASTER
  IP : STATE_BIO_MASTER/TACQ_BIO_MASTER
  GAS_BO_CTRL_Out : Outport
  GAS_MASK_Out : Outport  Port=2
  GAS_CTRL_Out : Outport  Port=3
  IP_BO_CTRL_Out : Outport  Port=4
  IP_MASK_Out : Outport  Port=5
  IP_CTRL_Out : Outport  Port=6
  wires:
  IP/2 -> IP_CTRL_Out/1
  GAS/1 -> GAS_MASK_Out/1
  IP_MON_In/1 -> IP/2
  IP/3 -> IP_BO_CTRL_Out/1
  GAS/2 -> GAS_CTRL_Out/1
  GAS/3 -> GAS_BO_CTRL_Out/1
  GAS_MON_In/1 -> GAS/2
  GAS_ISC_CTRL/1 -> GAS/1
  IP/1 -> IP_MASK_Out/1
  IP_ISC_CTRL/1 -> IP/1

== system TYPEB_MASTER/TYPEB_TOP_MASTER_shutdown/DACKILL_TYPEB ==
  note: AND is zero  (0) if all stages are OK
      | non-zero if BAD
  note: WDBLOCKFLAG is zero (0) if OK,
      | non-zero if BAD
  IP_WDBLOCKFLAG_In : Inport
  F0_WDBLOCKFLAG_In : Inport  Port=2
  F1_WDBLOCKFLAG_In : Inport  Port=3
  BF_WDBLOCKFLAG_In : Inport  Port=4
  IMTM_WDBLOCKFLAG_In : Inport  Port=5
  LogicalOperator1 : Logic  Operator=OR  Inputs=5  AllPortsSameDT=off  OutDataTypeStr=boolean
  STATE : cdsEpicsOut/Subsystem  Tag=cdsEpicsOutput  Description=|
      | Purpose:                                          
      | Output a FE signal to an EPICS channel.           
      |                                                   
      | Operation:                                        
      | Takes input value and passes it to EPICS record.  
      |                                                   
      | Usage:                                            
      | Name the part with the desired EPICS rrecord name.
      settings: AttributesFormatString=%<Tag>
  DACKILL_TRIG_Out : Outport
  wires:
  BF_WDBLOCKFLAG_In/1 -> LogicalOperator1/4
  IMTM_WDBLOCKFLAG_In/1 -> LogicalOperator1/5
  LogicalOperator1/1 -> STATE/1
  F1_WDBLOCKFLAG_In/1 -> LogicalOperator1/3
  F0_WDBLOCKFLAG_In/1 -> LogicalOperator1/2
  IP_WDBLOCKFLAG_In/1 -> LogicalOperator1/1
  STATE/1 -> DACKILL_TRIG_Out/1
